simulink model "FRUCD_VehicleSim_Model_V0_1_0"  (R2019b)
settings: Solver=VariableStepAuto  StartTime=0.0  StopTime=7.5  MaxStep=0.001  RelTol=1e-3
undefined symbols (not defined in the file): Alpha, Event, Kappa, Model, Parameter
settings Model: NumberOfSteps=2  Creator=bechr  LastModifiedBy=bechr
settings DebuggingCC: AllowedUnitSystems=CGS,SI,SI (extended)  UnderSpecifiedDimensionMsg=error
settings SFSimCC: CustomCodeUndefinedFunction=UseInterfaceOnly

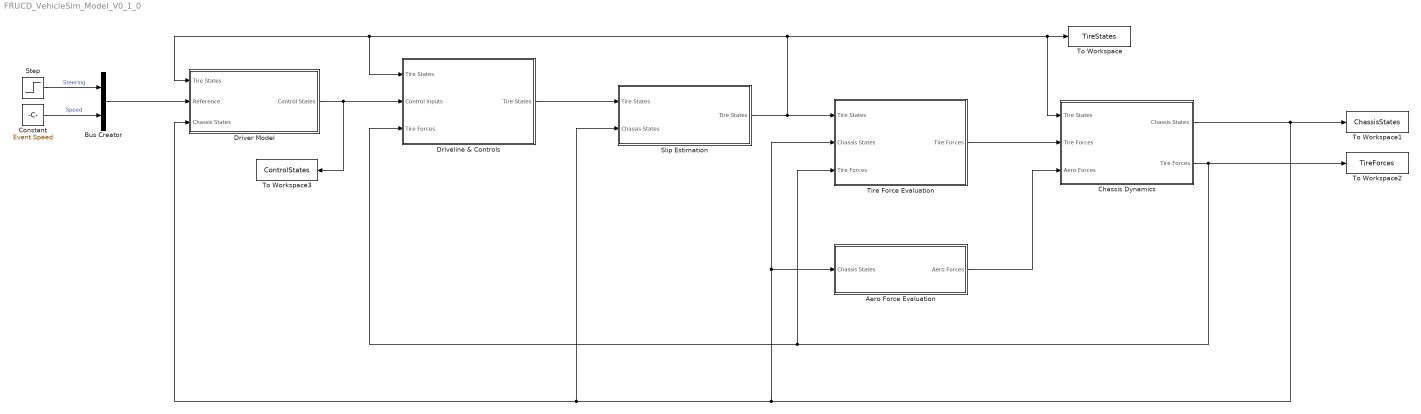
== system FRUCD_VehicleSim_Model_V0_1_0 ==
  Aero Force Evaluation : Subsystem
  Bus Creator : BusCreator  Inputs=2
  Chassis Dynamics : Subsystem  Variant=on
  Constant : Constant  Value=Event.Speed
  Driveline & Controls : Subsystem
  Driver Model : Subsystem  Variant=on
  Slip Estimation : Subsystem  Variant=on
  Step : Step  Time=0.2  After=Event.Amplitude  SampleTime=0
  Tire Force Evaluation : Subsystem
  To Workspace : ToWorkspace  VariableName=TireStates  SaveFormat=Timeseries  SampleTime=-1
  To Workspace1 : ToWorkspace  VariableName=ChassisStates  SaveFormat=Timeseries  SampleTime=-1
  To Workspace2 : ToWorkspace  VariableName=TireForces  SaveFormat=Timeseries  SampleTime=-1
  To Workspace3 : ToWorkspace  VariableName=ControlStates  SaveFormat=Timeseries  SampleTime=-1
  wires:
  Slip Estimation/1(" Tire States") -> Driver Model/1(Tire States), Driveline & Controls/1("Tire States "), To Workspace/1, Chassis Dynamics/1(Tire States), Tire Force Evaluation/1(Tire States)
  Driveline & Controls/1(Tire States) -> Slip Estimation/1(Tire States)
  Tire Force Evaluation/1(" Tire Forces") -> Chassis Dynamics/2("Tire Forces ")
  Chassis Dynamics/1(Chassis States) -> To Workspace1/1, Driver Model/3(Chassis States), Slip Estimation/2(Chassis States), Aero Force Evaluation/1(Chassis States), Tire Force Evaluation/2(Chassis States)
  Aero Force Evaluation/1(Aero Forces) -> Chassis Dynamics/3(Aero Forces)
  Driver Model/1(Control States) -> To Workspace3/1, Driveline & Controls/2(Control Inputs)
  Chassis Dynamics/2(" Tire Forces") -> To Workspace2/1, Driveline & Controls/3(Tire Forces), Tire Force Evaluation/3(Tire Forces)
  Step/1 -> Bus Creator/1  "Steering"
  Constant/1 -> Bus Creator/2  "Speed"
  Bus Creator/1 -> Driver Model/2(Reference)

== system FRUCD_VehicleSim_Model_V0_1_0/Aero Force Evaluation ==
  Chassis States : Inport
  Constant : Constant  Value=[0 0 0 0 0 0]
  Terminator : Terminator
  Aero Forces : Outport
  wires:
  Constant/1 -> Aero Forces/1
  Chassis States/1 -> Terminator/1

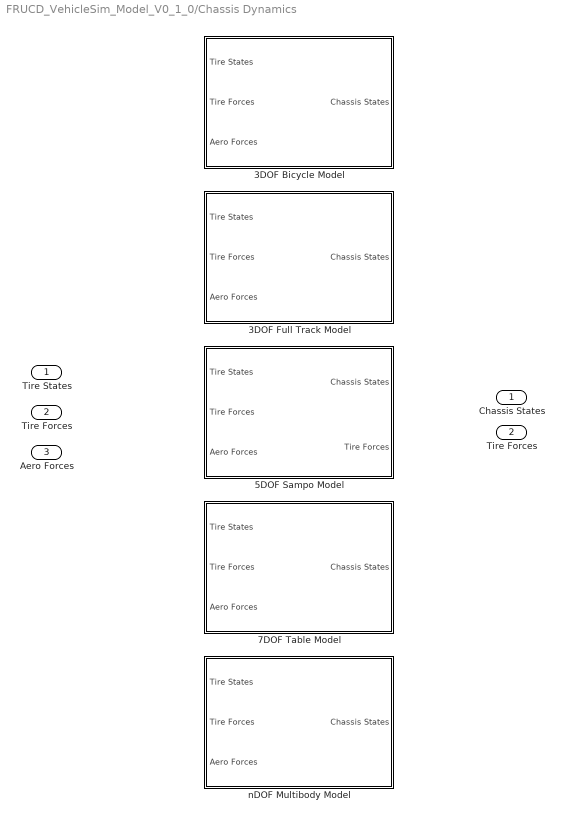
== system FRUCD_VehicleSim_Model_V0_1_0/Chassis Dynamics ==
  Tire States : Inport
  "Tire Forces " : Inport  Port=2
  Aero Forces : Inport  Port=3
  3DOF Bicycle Model : Subsystem  VariantControl="strcmp(Model.ChassisDynamics,\"3DOF Bicycle\")"
  3DOF Full Track Model : Subsystem  VariantControl="strcmp(Model.ChassisDynamics,\"3DOF Full Track\")"
  5DOF Sampo Model : Subsystem  VariantControl="strcmp(Model.ChassisDynamics,\"5DOF Sampo\")"
  "7DOF Table Model " : Subsystem  VariantControl="strcmp(Model.ChassisDynamics,\"7DOF Table\")"
  nDOF Multibody Model : Subsystem  VariantControl="strcmp(Model.ChassisDynamics,\"nDOF Multibody\")"
  Chassis States : Outport
  " Tire Forces" : Outport  Port=2

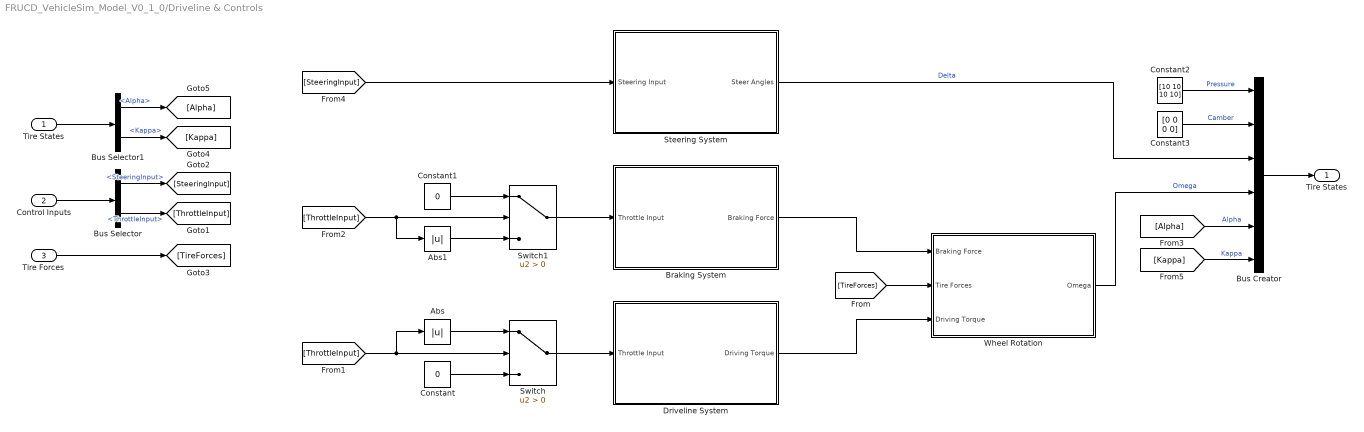
== system FRUCD_VehicleSim_Model_V0_1_0/Driveline & Controls ==
  "Tire States " : Inport
  Control Inputs : Inport  Port=2
  Tire Forces : Inport  Port=3
  Abs : Abs
  Abs1 : Abs
  Braking System : Subsystem  Variant=on
  Bus Creator : BusCreator  Inputs=6
  Bus Selector : BusSelector  OutputSignals=SteeringInput,ThrottleInput
  Bus Selector1 : BusSelector  OutputSignals=Alpha,Kappa
  Constant : Constant  Value=0
  Constant1 : Constant  Value=0
  Constant2 : Constant  Value=[10 10 10 10]
  Constant3 : Constant  Value=[0 0 0 0]
  Driveline System : Subsystem  Variant=on
  Steering System : Subsystem  Variant=on
  Switch : Switch  Criteria=u2 > Threshold
  Switch1 : Switch  Criteria=u2 > Threshold
  Wheel Rotation : Subsystem  Variant=on
  Tire States : Outport
  wires:
  Braking System/1(Braking Force) -> Wheel Rotation/1(Braking Force)
  Driveline System/1(Driving Torque) -> Wheel Rotation/3(Driving Torque)
  Tire Forces/1 -> [TireForces]
  [TireForces] -> Wheel Rotation/2(Tire Forces)
  Control Inputs/1 -> Bus Selector/1
  Bus Selector/1 -> [SteeringInput]  "<SteeringInput>"
  Bus Selector/2 -> [ThrottleInput]  "<ThrottleInput>"
  [ThrottleInput] -> Switch/2, Abs/1
  Switch/1 -> Driveline System/1(Throttle Input)
  Constant/1 -> Switch/3
  Abs/1 -> Switch/1
  Switch1/1 -> Braking System/1(Throttle Input)
  [ThrottleInput] -> Abs1/1, Switch1/2
  Constant1/1 -> Switch1/1
  Abs1/1 -> Switch1/3
  Bus Creator/1 -> Tire States/1
  Constant2/1 -> Bus Creator/1  "Pressure"
  Constant3/1 -> Bus Creator/2  "Camber"
  Wheel Rotation/1(Omega) -> Bus Creator/4  "Omega"
  Steering System/1(Steer Angles) -> Bus Creator/3  "Delta"
  [SteeringInput] -> Steering System/1(Steering Input)
  Bus Selector1/1 -> [Alpha]  "<Alpha>"
  Bus Selector1/2 -> [Kappa]  "<Kappa>"
  "Tire States "/1 -> Bus Selector1/1
  [Alpha] -> Bus Creator/5  "Alpha"
  [Kappa] -> Bus Creator/6  "Kappa"

== system FRUCD_VehicleSim_Model_V0_1_0/Driver Model ==
  Tire States : Inport
  Reference : Inport  Port=2
  Chassis States : Inport  Port=3
  MPC Path Following : Subsystem  VariantControl="strcmp(Model.Driver,\"Path Following\")"
  Open Loop Steer & Speed Regulation : Subsystem  VariantControl="strcmp(Model.Driver,\"Open Loop & Regulation Control\")"
  Control States : Outport

== system FRUCD_VehicleSim_Model_V0_1_0/Slip Estimation ==
  Tire States : Inport
  Chassis States : Inport  Port=2
  Full Fidelity : Subsystem  VariantControl="strcmp(Model.SlipEstimation,\"Full Fidelity\")"
  Planar Geometry : Subsystem  VariantControl="strcmp(Model.SlipEstimation,\"Planar\")"
  " Tire States" : Outport

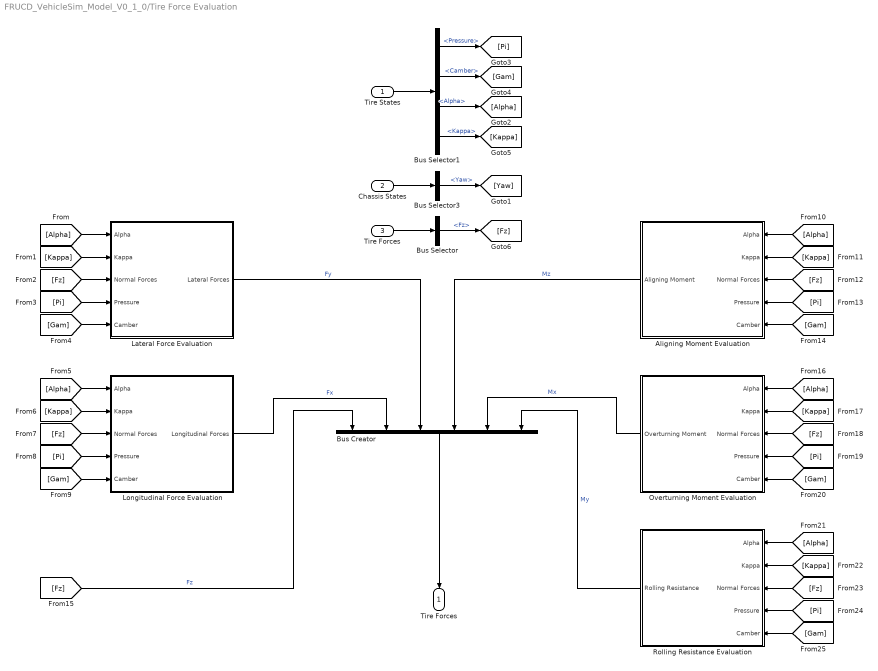
== system FRUCD_VehicleSim_Model_V0_1_0/Tire Force Evaluation ==
  Tire States : Inport
  Chassis States : Inport  Port=2
  Tire Forces : Inport  Port=3
  Aligning Moment Evaluation : Subsystem  Variant=on
  Bus Creator : BusCreator  Inputs=6
  Bus Selector : BusSelector  OutputSignals=Fz
  Bus Selector1 : BusSelector  OutputSignals=Pressure,Camber,Alpha,Kappa
  Bus Selector3 : BusSelector  OutputSignals=Vel.Yaw
  Lateral Force Evaluation : Subsystem  Variant=on
  Longitudinal Force Evaluation : Subsystem  Variant=on
  Overturning Moment Evaluation : Subsystem  Variant=on
  Rolling Resistance Evaluation : Subsystem  Variant=on
  " Tire Forces" : Outport  VectorParamsAs1DForOutWhenUnconnected=off
  wires:
  [Pi] -> Lateral Force Evaluation/4(Pressure)
  Bus Creator/1 -> " Tire Forces"/1
  Aligning Moment Evaluation/1(Aligning Moment) -> Bus Creator/4  "Mz"
  [Alpha] -> Aligning Moment Evaluation/1(Alpha)
  Rolling Resistance Evaluation/1(Rolling Resistance) -> Bus Creator/6  "My"
  [Fz] -> Bus Creator/1  "Fz"
  Longitudinal Force Evaluation/1(Longitudinal Forces) -> Bus Creator/2  "Fx"
  [Fz] -> Rolling Resistance Evaluation/3(Normal Forces)
  [Kappa] -> Longitudinal Force Evaluation/2(Kappa)
  [Pi] -> Rolling Resistance Evaluation/4(Pressure)
  [Gam] -> Overturning Moment Evaluation/5(Camber)
  Overturning Moment Evaluation/1(Overturning Moment) -> Bus Creator/5  "Mx"
  [Kappa] -> Lateral Force Evaluation/2(Kappa)
  Lateral Force Evaluation/1(Lateral Forces) -> Bus Creator/3  "Fy"
  [Kappa] -> Rolling Resistance Evaluation/2(Kappa)
  [Alpha] -> Lateral Force Evaluation/1(Alpha)
  [Gam] -> Rolling Resistance Evaluation/5(Camber)
  [Fz] -> Lateral Force Evaluation/3(Normal Forces)
  [Fz] -> Aligning Moment Evaluation/3(Normal Forces)
  [Fz] -> Overturning Moment Evaluation/3(Normal Forces)
  [Pi] -> Longitudinal Force Evaluation/4(Pressure)
  [Pi] -> Overturning Moment Evaluation/4(Pressure)
  [Alpha] -> Overturning Moment Evaluation/1(Alpha)
  [Kappa] -> Overturning Moment Evaluation/2(Kappa)
  [Pi] -> Aligning Moment Evaluation/4(Pressure)
  [Gam] -> Lateral Force Evaluation/5(Camber)
  [Alpha] -> Longitudinal Force Evaluation/1(Alpha)
  [Kappa] -> Aligning Moment Evaluation/2(Kappa)
  [Gam] -> Aligning Moment Evaluation/5(Camber)
  [Fz] -> Longitudinal Force Evaluation/3(Normal Forces)
  [Gam] -> Longitudinal Force Evaluation/5(Camber)
  [Alpha] -> Rolling Resistance Evaluation/1(Alpha)
  Tire Forces/1 -> Bus Selector/1
  Bus Selector/1 -> [Fz]  "<Fz>"
  Tire States/1 -> Bus Selector1/1
  Bus Selector1/2 -> [Gam]  "<Camber>"
  Bus Selector1/1 -> [Pi]  "<Pressure>"
  Chassis States/1 -> Bus Selector3/1
  Bus Selector3/1 -> [Yaw]  "<Yaw>"
  Bus Selector1/3 -> [Alpha]  "<Alpha>"
  Bus Selector1/4 -> [Kappa]  "<Kappa>"

== system FRUCD_VehicleSim_Model_V0_1_0/Chassis Dynamics/3DOF Bicycle Model ==
  Tire States : Inport
  "Tire Forces " : Inport  Port=2
  Aero Forces : Inport  Port=3
  Chassis States : Outport

== system FRUCD_VehicleSim_Model_V0_1_0/Chassis Dynamics/3DOF Full Track Model ==
  Tire States : Inport
  "Tire Forces " : Inport  Port=2
  Aero Forces : Inport  Port=3
  Chassis States : Outport

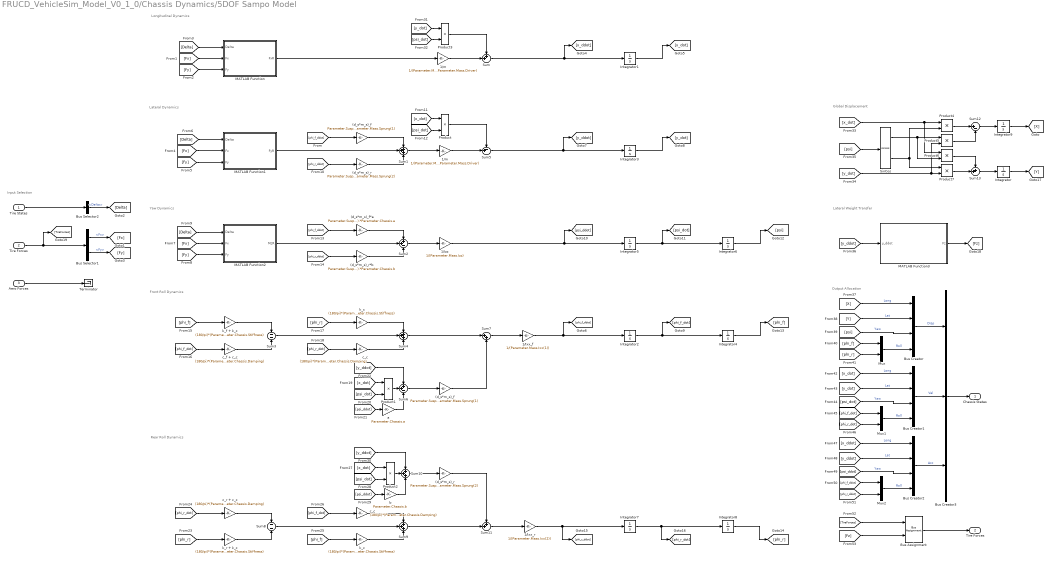
== system FRUCD_VehicleSim_Model_V0_1_0/Chassis Dynamics/5DOF Sampo Model ==
  note: Output Allocation
  note: Lateral Weight Transfer
  note: Global Displacement
  note: Input Selection
  note: Rear Roll Dynamics
  note: Front Roll Dynamics
  note: Yaw Dynamics
  note: Lateral Dynamics
  note: Longitudinal Dynamics
  Tire States : Inport
  "Tire Forces " : Inport  Port=2
  Aero Forces : Inport  Port=3
  (d_s*m_s)_f : Gain  Gain=Parameter.Suspension.Roll.Arm(1).*Parameter.Mass.Sprung(1)
  "(d_s*m_s)_f " : Gain  Gain=Parameter.Suspension.Roll.Arm(1).*Parameter.Mass.Sprung(1)
  (d_s*m_s)_f*a : Gain  Gain=Parameter.Suspension.Roll.Arm(1).*Parameter.Mass.Sprung(1).*Parameter.Chassis.a
  (d_s*m_s)_r : Gain  Gain=Parameter.Suspension.Roll.Arm(2).*Parameter.Mass.Sprung(2)
  "(d_s*m_s)_r " : Gain  Gain=Parameter.Suspension.Roll.Arm(2).*Parameter.Mass.Sprung(2)
  (d_s*m_s)_r*b : Gain  Gain=Parameter.Suspension.Roll.Arm(2).*Parameter.Mass.Sprung(2).*Parameter.Chassis.b
  1/Ixx_f : Gain  Gain=1/(Parameter.Mass.Ixx(1))
  1/Ixx_r : Gain  Gain=1/(Parameter.Mass.Ixx(2))
  1/Izz : Gain  Gain=1/(Parameter.Mass.Izz)
  1/m : Gain  Gain=1/(Parameter.Mass.Vehicle+Parameter.Mass.Driver)
  "1/m " : Gain  Gain=1/(Parameter.Mass.Vehicle+Parameter.Mass.Driver)
  Bus Assignment : BusAssignment  AssignedSignals=Fz
  Bus Creator : BusCreator  Inputs=4
  Bus Creator1 : BusCreator  Inputs=4
  Bus Creator2 : BusCreator  Inputs=4
  Bus Creator3 : BusCreator  Inputs=3
  Bus Selector1 : BusSelector  OutputSignals=Fx,Fy
  Bus Selector2 : BusSelector  OutputSignals=Delta
  Integrator{,2..9} (9 alike) : Integrator
  Integrator1 : Integrator  InitialCondition=Event.Speed
  MATLAB Function : MATLAB Function  TreatAsAtomicUnit=on
  MATLAB Function1 : MATLAB Function  TreatAsAtomicUnit=on
  MATLAB Function2 : MATLAB Function  TreatAsAtomicUnit=on
  MATLAB Function3 : MATLAB Function  TreatAsAtomicUnit=on
  Mux : Mux  Inputs=2
  Mux1 : Mux  Inputs=2
  Mux2 : Mux  Inputs=2
  Product{,1..7} (8 alike) : Product
  SinCos : Trigonometry  Operator=sincos
  Sum : Sum  Inputs=++|
  Sum{1,4,9..10} (4 alike) : Sum  Inputs=+++
  Sum11 : Sum  Inputs=++|
  Sum12 : Sum  Inputs=|+-
  Sum13 : Sum  Inputs=++|
  Sum2 : Sum  Inputs=++-
  Sum3 : Sum  Inputs=-|-
  Sum5 : Sum  Inputs=-+|
  Sum6 : Sum  Inputs=++-
  Sum7 : Sum  Inputs=|++
  Sum8 : Sum  Inputs=-|-
  Terminator : Terminator
  a : Gain  Gain=Parameter.Chassis.a
  b : Gain  Gain=Parameter.Chassis.b
  c_c : Gain  Gain=(180/pi)*(Parameter.Chassis.Damping)
  "c_c " : Gain  Gain=(180/pi)*(Parameter.Chassis.Damping)
  c_f + c_c : Gain  Gain=(180/pi)*(Parameter.Suspension.Roll.Damping(1)+Parameter.Chassis.Damping)
  c_r + c_c : Gain  Gain=(180/pi)*(Parameter.Suspension.Roll.Damping(2)+Parameter.Chassis.Damping)
  k_c : Gain  Gain=(180/pi)*(Parameter.Chassis.Stiffness)
  "k_c " : Gain  Gain=(180/pi)*(Parameter.Chassis.Stiffness)
  k_f + k_c : Gain  Gain=(180/pi)*(Parameter.Suspension.Roll.Stiffness(1)+Parameter.Chassis.Stiffness)
  k_r + k_c : Gain  Gain=(180/pi)*(Parameter.Suspension.Roll.Stiffness(2)+Parameter.Chassis.Stiffness)
  Chassis States : Outport
  " Tire Forces" : Outport  Port=2
  wires:
  Tire States/1 -> Bus Selector2/1
  Bus Selector2/1 -> [Delta]  "<Delta>"
  Bus Selector1/2 -> [Fy]  "<Fy>"
  Bus Selector1/1 -> [Fx]  "<Fx>"
  Aero Forces/1 -> Terminator/1
  Product3/1 -> Sum/1
  c_f + c_c/1 -> Sum3/2
  [psi_dot] -> Product2/2
  "c_c "/1 -> Sum9/1
  Sum6/1 -> "(d_s*m_s)_f "/1
  [psi_dot] -> Product3/2
  b/1 -> Sum10/3
  MATLAB Function1/1(FyR) -> Sum1/2
  Integrator7/1 -> [phi_r_dot], Integrator8/1
  [phi_f_ddot] -> (d_s*m_s)_f*a/1
  Sum7/1 -> 1/Ixx_f/1
  [Delta] -> MATLAB Function1/1(Delta)
  Sum1/1 -> "1/m "/1
  Sum11/1 -> 1/Ixx_r/1
  "(d_s*m_s)_f "/1 -> Sum7/2
  [y_ddot] -> Sum10/1
  [psi_dot] -> Product1/2
  [psi_dot] -> Product/2
  [phi_r] -> k_c/1
  "k_c "/1 -> Sum9/3
  Product2/1 -> Sum10/2
  Sum8/1 -> Sum9/2
  [phi_f_dot] -> c_f + c_c/1
  Product1/1 -> Sum6/2
  [phi_r] -> k_r + k_c/1
  MATLAB Function2/1(MzR) -> Sum2/2
  [Fx] -> MATLAB Function2/2(Fx)
  [phi_f_dot] -> "c_c "/1
  [phi_r_dot] -> c_c/1
  [x_dot] -> Product1/1
  [psi_ddot] -> a/1
  "1/m "/1 -> Sum5/2
  [Fy] -> MATLAB Function2/3(Fy)
  [phi_r_ddot] -> (d_s*m_s)_r*b/1
  1/Izz/1 -> [psi_ddot], Integrator5/1
  [x_dot] -> Product2/1
  Integrator5/1 -> [psi_dot], Integrator6/1
  Integrator4/1 -> [phi_f]
  [phi_f_ddot] -> (d_s*m_s)_f/1
  Sum4/1 -> Sum7/1
  c_r + c_c/1 -> Sum8/1
  [x_dot] -> Product/1
  Sum2/1 -> 1/Izz/1
  [phi_f] -> k_f + k_c/1
  "(d_s*m_s)_r "/1 -> Sum11/1
  Sum9/1 -> Sum11/2
  [y_ddot] -> Sum6/1
  (d_s*m_s)_r/1 -> Sum1/3
  [Fy] -> MATLAB Function/3(Fy)
  Integrator3/1 -> [y_dot]
  Product/1 -> Sum5/1
  Integrator1/1 -> [x_dot]
  MATLAB Function/1(FxR) -> 1/m/1
  1/m/1 -> Sum/2
  (d_s*m_s)_f/1 -> Sum1/1
  Integrator8/1 -> [phi_r]
  (d_s*m_s)_f*a/1 -> Sum2/1
  Sum3/1 -> Sum4/2
  Integrator6/1 -> [psi]
  1/Ixx_r/1 -> [phi_r_ddot], Integrator7/1
  Sum10/1 -> "(d_s*m_s)_r "/1
  Integrator2/1 -> [phi_f_dot], Integrator4/1
  a/1 -> Sum6/3
  k_f + k_c/1 -> Sum3/1
  c_c/1 -> Sum4/3
  1/Ixx_f/1 -> [phi_f_ddot], Integrator2/1
  Sum/1 -> [x_ddot], Integrator1/1
  [psi_ddot] -> b/1
  [y_dot] -> Product3/1
  (d_s*m_s)_r*b/1 -> Sum2/3
  [Fx] -> MATLAB Function1/2(Fx)
  k_c/1 -> Sum4/1
  k_r + k_c/1 -> Sum8/2
  [Delta] -> MATLAB Function/1(Delta)
  Sum5/1 -> [y_ddot], Integrator3/1
  [Fx] -> MATLAB Function/2(Fx)
  [phi_r_ddot] -> (d_s*m_s)_r/1
  [phi_f] -> "k_c "/1
  [Fy] -> MATLAB Function1/3(Fy)
  [phi_r_dot] -> c_r + c_c/1
  [Delta] -> MATLAB Function2/1(Delta)
  [x_dot] -> Product4/1, Product6/1
  [y_dot] -> Product5/2, Product7/2
  SinCos/1 -> Product6/2, Product5/1
  SinCos/2 -> Product7/1, Product4/2
  Product4/1 -> Sum12/1
  Product5/1 -> Sum12/2
  Product6/1 -> Sum13/1
  Product7/1 -> Sum13/2
  Sum13/1 -> Integrator/1
  Sum12/1 -> Integrator9/1
  Integrator9/1 -> [X]
  Integrator/1 -> [Y]
  [y_ddot] -> MATLAB Function3/1(y_ddot)
  MATLAB Function3/1(Fz) -> [Fz]
  [phi_f] -> Mux/1
  [phi_r] -> Mux/2
  [X] -> Bus Creator/1  "Long"
  [Y] -> Bus Creator/2  "Lat"
  [psi] -> Bus Creator/3  "Yaw"
  Mux/1 -> Bus Creator/4  "Roll"
  [phi_f_dot] -> Mux1/1
  [psi_dot] -> Bus Creator1/3  "Yaw"
  [phi_r_dot] -> Mux1/2
  [y_dot] -> Bus Creator1/2  "Lat"
  Mux1/1 -> Bus Creator1/4  "Roll"
  [x_dot] -> Bus Creator1/1  "Long"
  [psi_ddot] -> Bus Creator2/3  "Yaw"
  [phi_r_ddot] -> Mux2/2
  [phi_f_ddot] -> Mux2/1
  [x_ddot] -> Bus Creator2/1  "Long"
  Mux2/1 -> Bus Creator2/4  "Roll"
  [y_ddot] -> Bus Creator2/2  "Lat"
  Bus Creator2/1 -> Bus Creator3/3  "Acc"
  Bus Creator1/1 -> Bus Creator3/2  "Vel"
  Bus Creator/1 -> Bus Creator3/1  "Disp"
  Bus Creator3/1 -> Chassis States/1
  "Tire Forces "/1 -> [TireForces], Bus Selector1/1
  [TireForces] -> Bus Assignment/1
  [Fz] -> Bus Assignment/2
  Bus Assignment/1 -> " Tire Forces"/1
  [psi] -> SinCos/1

== system FRUCD_VehicleSim_Model_V0_1_0/Chassis Dynamics/7DOF Table Model  ==
  Tire States : Inport
  "Tire Forces " : Inport  Port=2
  Aero Forces : Inport  Port=3
  Chassis States : Outport

== system FRUCD_VehicleSim_Model_V0_1_0/Chassis Dynamics/nDOF Multibody Model ==
  Tire States : Inport
  "Tire Forces " : Inport  Port=2
  Aero Forces : Inport  Port=3
  Chassis States : Outport

== system FRUCD_VehicleSim_Model_V0_1_0/Driveline & Controls/Braking System ==
  Throttle Input : Inport
  Bond Graph Model : Subsystem  VariantControl="strcmp(Model.BrakingSystem,\"Bond Graph Model\")"
  Linear Gains : Subsystem  VariantControl="strcmp(Model.BrakingSystem,\"Simple Gains\")"
  Braking Force : Outport

== system FRUCD_VehicleSim_Model_V0_1_0/Driveline & Controls/Driveline System ==
  Throttle Input : Inport
  Bond Graph : Subsystem  VariantControl="strcmp(Model.DrivelineSystem,\"Bond Graph Model\")"
  Linear Gains : Subsystem  VariantControl="strcmp(Model.DrivelineSystem,\"Simple Gains\")"
  Driving Torque : Outport

== system FRUCD_VehicleSim_Model_V0_1_0/Driveline & Controls/Steering System ==
  Steering Input : Inport
  Ackermann Lookup : Subsystem  VariantControl="strcmp(Model.SteeringSystem,\"Lookup Table\")"
  Linear Gain : Subsystem  VariantControl="strcmp(Model.SteeringSystem,\"Simple Gains\")"
  Steer Angles : Outport

== system FRUCD_VehicleSim_Model_V0_1_0/Driveline & Controls/Wheel Rotation ==
  Braking Force : Inport
  Tire Forces : Inport  Port=2
  Driving Torque : Inport  Port=3
  Simple ODE : Subsystem  VariantControl="strcmp(Model.WheelRotation,\"Simple ODE\")"
  Omega : Outport

== system FRUCD_VehicleSim_Model_V0_1_0/Driver Model/MPC Path Following ==
  Tire States : Inport
  Reference : Inport  Port=2
  Chassis States : Inport  Port=3
  Control States : Outport

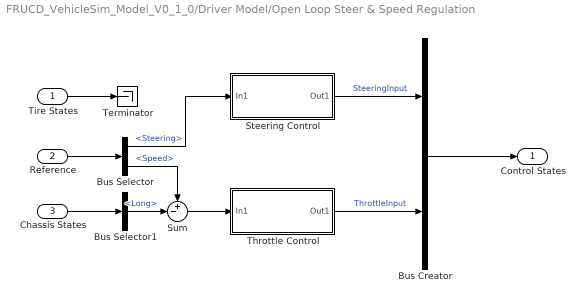
== system FRUCD_VehicleSim_Model_V0_1_0/Driver Model/Open Loop Steer & Speed Regulation ==
  Tire States : Inport
  Reference : Inport  Port=2
  Chassis States : Inport  Port=3
  Bus Creator : BusCreator  Inputs=2
  Bus Selector : BusSelector  OutputSignals=Steering,Speed
  Bus Selector1 : BusSelector  OutputSignals=Vel.Long
  Steering Control : Subsystem
  Sum : Sum  Inputs=+-|
  Terminator : Terminator
  Throttle Control : Subsystem
  Control States : Outport
  wires:
  Reference/1 -> Bus Selector/1
  Tire States/1 -> Terminator/1
  Chassis States/1 -> Bus Selector1/1
  Steering Control/1(Out1) -> Bus Creator/1  "SteeringInput"
  Throttle Control/1(Out1) -> Bus Creator/2  "ThrottleInput"
  Bus Creator/1 -> Control States/1
  Bus Selector/1 -> Steering Control/1(In1)  "<Steering>"
  Bus Selector/2 -> Sum/1  "<Speed>"
  Bus Selector1/1 -> Sum/2  "<Long>"
  Sum/1 -> Throttle Control/1(In1)

== system FRUCD_VehicleSim_Model_V0_1_0/Slip Estimation/Full Fidelity ==
  Chassis States : Inport
  Tire States : Inport  Port=2
  " Tire States" : Outport

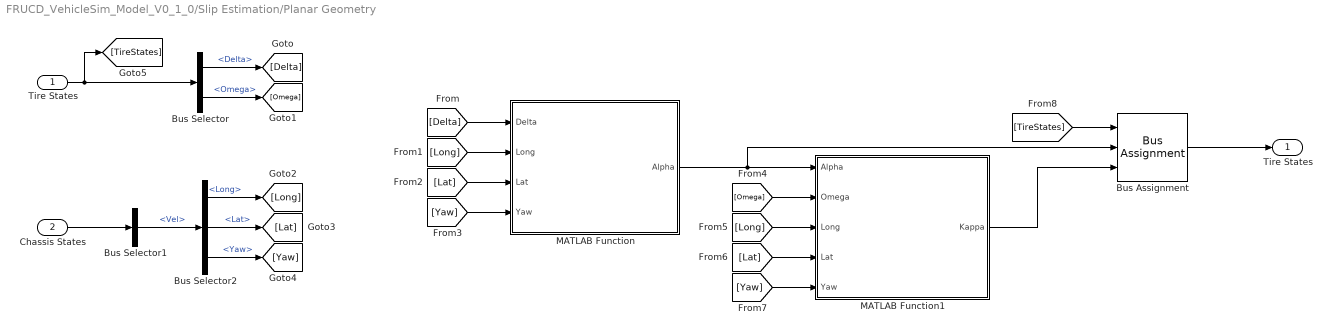
== system FRUCD_VehicleSim_Model_V0_1_0/Slip Estimation/Planar Geometry ==
  Tire States : Inport
  Chassis States : Inport  Port=2
  Bus Assignment : BusAssignment  AssignedSignals=Alpha,Kappa
  Bus Selector : BusSelector  OutputSignals=Delta,Omega
  Bus Selector1 : BusSelector  OutputSignals=Vel
  Bus Selector2 : BusSelector  OutputSignals=Long,Lat,Yaw
  MATLAB Function : MATLAB Function  TreatAsAtomicUnit=on
  MATLAB Function1 : MATLAB Function  TreatAsAtomicUnit=on
  " Tire States" : Outport
  wires:
  [Yaw] -> MATLAB Function/4(Yaw)
  [Lat] -> MATLAB Function/3(Lat)
  [Long] -> MATLAB Function/2(Long)
  [Delta] -> MATLAB Function/1(Delta)
  Tire States/1 -> [TireStates], Bus Selector/1
  [Yaw] -> MATLAB Function1/5(Yaw)
  [Lat] -> MATLAB Function1/4(Lat)
  [Long] -> MATLAB Function1/3(Long)
  [Omega] -> MATLAB Function1/2(Omega)
  MATLAB Function/1(Alpha) -> Bus Assignment/2, MATLAB Function1/1(Alpha)
  Bus Selector/1 -> [Delta]  "<Delta>"
  Bus Selector/2 -> [Omega]  "<Omega>"
  Chassis States/1 -> Bus Selector1/1
  [TireStates] -> Bus Assignment/1
  Bus Assignment/1 -> " Tire States"/1
  Bus Selector1/1 -> Bus Selector2/1  "<Vel>"
  Bus Selector2/1 -> [Long]  "<Long>"
  Bus Selector2/2 -> [Lat]  "<Lat>"
  Bus Selector2/3 -> [Yaw]  "<Yaw>"
  MATLAB Function1/1(Kappa) -> Bus Assignment/3

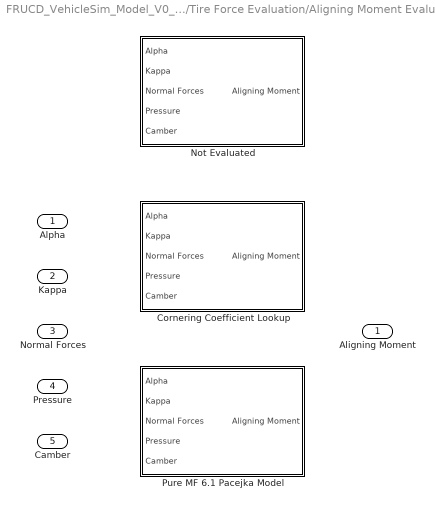
== system FRUCD_VehicleSim_Model_V0_1_0/Tire Force Evaluation/Aligning Moment Evaluation ==
  Alpha : Inport
  Kappa : Inport  Port=2
  Normal Forces : Inport  Port=3
  Pressure : Inport  Port=4
  Camber : Inport  Port=5
  Cornering Coefficient Lookup : Subsystem  VariantControl="strcmp(Model.TireForceEvaluation.Aligning,\"Cornering Coefficient\")"
  Not Evaluated : Subsystem  VariantControl="strcmp(Model.TireForceEvaluation.Aligning,\"Not Evaluated\")"
  Pure MF 6.1 Pacejka Model : Subsystem  VariantControl="strcmp(Model.TireForceEvaluation.Aligning,\"Pure MF6.1\")"
  Aligning Moment : Outport  VectorParamsAs1DForOutWhenUnconnected=off

== system FRUCD_VehicleSim_Model_V0_1_0/Tire Force Evaluation/Lateral Force Evaluation ==
  Alpha : Inport
  Kappa : Inport  Port=2
  Normal Forces : Inport  Port=3
  Pressure : Inport  Port=4
  Camber : Inport  Port=5
  Cornering Coefficient Lookup : Subsystem  VariantControl="strcmp(Model.TireForceEvaluation.Lateral,\"Cornering Coefficient\")"
  Pure MF 6.1 Pacejka Model : Subsystem  VariantControl="strcmp(Model.TireForceEvaluation.Lateral,\"Pure MF6.1\")"
  Lateral Forces : Outport  VectorParamsAs1DForOutWhenUnconnected=off

== system FRUCD_VehicleSim_Model_V0_1_0/Tire Force Evaluation/Longitudinal Force Evaluation ==
  Alpha : Inport
  Kappa : Inport  Port=2
  Normal Forces : Inport  Port=3
  Pressure : Inport  Port=4
  Camber : Inport  Port=5
  Cornering Coefficient Lookup : Subsystem  VariantControl="strcmp(Model.TireForceEvaluation.Longitudinal,\"Cornering Coefficient\")"
  Pure MF 6.1 Pacejka Model : Subsystem  VariantControl="strcmp(Model.TireForceEvaluation.Longitudinal,\"Pure MF6.1\")"
  Longitudinal Forces : Outport  VectorParamsAs1DForOutWhenUnconnected=off

== system FRUCD_VehicleSim_Model_V0_1_0/Tire Force Evaluation/Overturning Moment Evaluation ==
  Alpha : Inport
  Kappa : Inport  Port=2
  Normal Forces : Inport  Port=3
  Pressure : Inport  Port=4
  Camber : Inport  Port=5
  Cornering Coefficient Lookup : Subsystem  VariantControl="strcmp(Model.TireForceEvaluation.Overturning,\"Cornering Coefficient\")"
  Not Evaluated : Subsystem  VariantControl="strcmp(Model.TireForceEvaluation.Overturning,\"Not Evaluated\")"
  Pure MF 6.1 Pacejka Model : Subsystem  VariantControl="strcmp(Model.TireForceEvaluation.Overturning,\"Pure MF6.1\")"
  Overturning Moment : Outport  VectorParamsAs1DForOutWhenUnconnected=off

== system FRUCD_VehicleSim_Model_V0_1_0/Tire Force Evaluation/Rolling Resistance Evaluation ==
  Alpha : Inport
  Kappa : Inport  Port=2
  Normal Forces : Inport  Port=3
  Pressure : Inport  Port=4
  Camber : Inport  Port=5
  Cornering Coefficient Lookup : Subsystem  VariantControl="strcmp(Model.TireForceEvaluation.Rolling,\"Cornering Coefficient\")"
  Not Evaluated : Subsystem  VariantControl="strcmp(Model.TireForceEvaluation.Overturning,\"Not Evaluated\")"
  Pure MF 6.1 Pacejka Model : Subsystem  VariantControl="strcmp(Model.TireForceEvaluation.Rolling,\"Pure MF6.1\")"
  Rolling Resistance : Outport  VectorParamsAs1DForOutWhenUnconnected=off

== system FRUCD_VehicleSim_Model_V0_1_0/Driveline & Controls/Braking System/Bond Graph Model ==
  Throttle Input : Inport
  Braking Force : Outport

== system FRUCD_VehicleSim_Model_V0_1_0/Driveline & Controls/Braking System/Linear Gains ==
  Throttle Input : Inport
  Friction Coefficient [ ] : Gain  Gain=Parameter.Brake.Pad.Mu
  Front Bore Area [m^2] : Gain  Gain=1 / (pi*Parameter.Brake.Cylinder.Bore(1)^2)
  Mux : Mux
  Pad Area [m^2] * Pad Quantity [ ] : Gain  Gain=Parameter.Brake.Pad.No*Parameter.Brake.Pad.Area
  Pedal Force [N] : Gain  Gain=Parameter.Brake.Pedal.Force
  Pedal Ratio [ ] : Gain  Gain=Parameter.Brake.Pedal.Ratio
  Rear Bore Area [m^2] : Gain  Gain=1 / (pi*Parameter.Brake.Cylinder.Bore(2)^2)
  Braking Force : Outport
  wires:
  Throttle Input/1 -> Pedal Force [N]/1
  Pedal Force [N]/1 -> Pedal Ratio [ ]/1
  Front Bore Area [m^2]/1 -> Mux/1, Mux/2
  Rear Bore Area [m^2]/1 -> Mux/3, Mux/4
  Mux/1 -> Pad Area [m^2] * Pad Quantity [ ]/1
  Pad Area [m^2] * Pad Quantity [ ]/1 -> Friction Coefficient [ ]/1
  Friction Coefficient [ ]/1 -> Braking Force/1
  Pedal Ratio [ ]/1 -> Front Bore Area [m^2]/1, Rear Bore Area [m^2]/1

== system FRUCD_VehicleSim_Model_V0_1_0/Driveline & Controls/Driveline System/Bond Graph ==
  Throttle Input : Inport
  Driving Torque : Outport

== system FRUCD_VehicleSim_Model_V0_1_0/Driveline & Controls/Driveline System/Linear Gains ==
  Throttle Input : Inport
  Constant : Constant  Value=0
  Maximum Torque [Nm] : Gain  Gain=157/2
  Mux : Mux
  Driving Torque : Outport
  wires:
  Throttle Input/1 -> Maximum Torque [Nm]/1
  Constant/1 -> Mux/2, Mux/1
  Maximum Torque [Nm]/1 -> Mux/4, Mux/3
  Mux/1 -> Driving Torque/1

== system FRUCD_VehicleSim_Model_V0_1_0/Driveline & Controls/Steering System/Ackermann Lookup ==
  Steering Input : Inport
  Steer Angles : Outport

== system FRUCD_VehicleSim_Model_V0_1_0/Driveline & Controls/Steering System/Linear Gain ==
  Steering Input : Inport
  Ackermann Lookup : Lookup_n-D  NumberOfTableDimensions=1  BreakpointsForDimension1=linspace(-120,120,20)  Table=linspace(-30,30,20)  InterpMethod=Cubic spline  InternalRulePriority=Speed  RndMeth=Simplest  InputSameDT=on
  Constant : Constant  Value=0
  Max Steering Angle [deg] : Gain  Gain=120
  Mux : Mux
  Steer Angles : Outport
  wires:
  Steering Input/1 -> Max Steering Angle [deg]/1
  Max Steering Angle [deg]/1 -> Ackermann Lookup/1
  Mux/1 -> Steer Angles/1
  Constant/1 -> Mux/4, Mux/3
  Ackermann Lookup/1 -> Mux/2, Mux/1

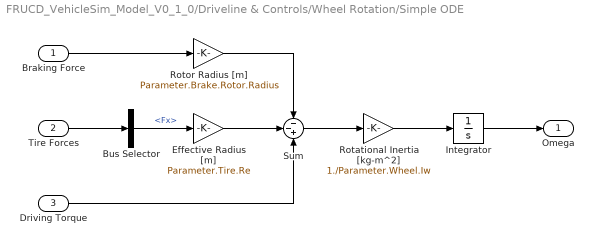
== system FRUCD_VehicleSim_Model_V0_1_0/Driveline & Controls/Wheel Rotation/Simple ODE ==
  Braking Force : Inport
  Tire Forces : Inport  Port=2
  Driving Torque : Inport  Port=3
  Bus Selector : BusSelector  OutputSignals=Fx
  Effective Radius [m] : Gain  Gain=Parameter.Tire.Re
  Integrator : Integrator  InitialCondition=Event.Speed/Parameter.Tire.Re.*ones(4,1)
  Rotational Inertia [kg-m^2] : Gain  Gain=1./Parameter.Wheel.Iw
  Rotor Radius [m] : Gain  Gain=Parameter.Brake.Rotor.Radius
  Sum : Sum  Inputs=--+
  Omega : Outport
  wires:
  Tire Forces/1 -> Bus Selector/1
  Effective Radius [m]/1 -> Sum/2
  Rotor Radius [m]/1 -> Sum/1
  Bus Selector/1 -> Effective Radius [m]/1  "<Fx>"
  Sum/1 -> Rotational Inertia [kg-m^2]/1
  Rotational Inertia [kg-m^2]/1 -> Integrator/1
  Integrator/1 -> Omega/1
  Braking Force/1 -> Rotor Radius [m]/1
  Driving Torque/1 -> Sum/3

== system FRUCD_VehicleSim_Model_V0_1_0/Driver Model/Open Loop Steer & Speed Regulation/Steering Control ==
  In1 : Inport
  Out1 : Outport
  wires:
  In1/1 -> Out1/1

== system FRUCD_VehicleSim_Model_V0_1_0/Driver Model/Open Loop Steer & Speed Regulation/Throttle Control ==
  In1 : Inport
  Saturation : Saturate  UpperLimit=1  LowerLimit=-1
  Out1 : Outport
  wires:
  Saturation/1 -> Out1/1
  In1/1 -> Saturation/1

== system FRUCD_VehicleSim_Model_V0_1_0/Tire Force Evaluation/Aligning Moment Evaluation/Cornering Coefficient Lookup ==
  Alpha : Inport
  Kappa : Inport  Port=2
  Normal Forces : Inport  Port=3
  Pressure : Inport  Port=4
  Camber : Inport  Port=5
  MATLAB Function : MATLAB Function  TreatAsAtomicUnit=on
  Aligning Moment : Outport  VectorParamsAs1DForOutWhenUnconnected=off
  wires:
  Camber/1 -> MATLAB Function/5(Gam)
  Pressure/1 -> MATLAB Function/4(Pi)
  Normal Forces/1 -> MATLAB Function/3(Fz)
  Kappa/1 -> MATLAB Function/2(unused)
  Alpha/1 -> MATLAB Function/1(a)
  MATLAB Function/1(Fyo) -> Aligning Moment/1

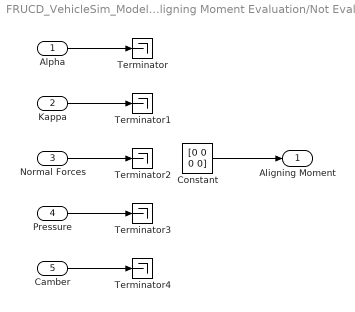
== system FRUCD_VehicleSim_Model_V0_1_0/Tire Force Evaluation/Aligning Moment Evaluation/Not Evaluated ==
  Alpha : Inport
  Kappa : Inport  Port=2
  Normal Forces : Inport  Port=3
  Pressure : Inport  Port=4
  Camber : Inport  Port=5
  Constant : Constant  Value=[0 0 0 0]
  Terminator{,1..4} (5 alike) : Terminator
  Aligning Moment : Outport  VectorParamsAs1DForOutWhenUnconnected=off
  wires:
  Kappa/1 -> Terminator1/1
  Alpha/1 -> Terminator/1
  Constant/1 -> Aligning Moment/1
  Normal Forces/1 -> Terminator2/1
  Pressure/1 -> Terminator3/1
  Camber/1 -> Terminator4/1

== system FRUCD_VehicleSim_Model_V0_1_0/Tire Force Evaluation/Aligning Moment Evaluation/Pure MF 6.1 Pacejka Model ==
  Alpha : Inport
  Kappa : Inport  Port=2
  Normal Forces : Inport  Port=3
  Pressure : Inport  Port=4
  Camber : Inport  Port=5
  MATLAB Function : MATLAB Function  TreatAsAtomicUnit=on
  Aligning Moment : Outport  VectorParamsAs1DForOutWhenUnconnected=off
  wires:
  MATLAB Function/1(Fyo) -> Aligning Moment/1
  Alpha/1 -> MATLAB Function/1(Alpha)
  Kappa/1 -> MATLAB Function/2(unused)
  Normal Forces/1 -> MATLAB Function/3(Fz)
  Pressure/1 -> MATLAB Function/4(Pi)
  Camber/1 -> MATLAB Function/5(Gam)

== system FRUCD_VehicleSim_Model_V0_1_0/Tire Force Evaluation/Lateral Force Evaluation/Cornering Coefficient Lookup ==
  Alpha : Inport
  Kappa : Inport  Port=2
  Normal Forces : Inport  Port=3
  Pressure : Inport  Port=4
  Camber : Inport  Port=5
  MATLAB Function : MATLAB Function  TreatAsAtomicUnit=on
  Lateral Forces : Outport  VectorParamsAs1DForOutWhenUnconnected=off
  wires:
  Camber/1 -> MATLAB Function/5(Gam)
  Pressure/1 -> MATLAB Function/4(Pi)
  Normal Forces/1 -> MATLAB Function/3(Fz)
  Kappa/1 -> MATLAB Function/2(unused)
  Alpha/1 -> MATLAB Function/1(Alpha)
  MATLAB Function/1(Fyo) -> Lateral Forces/1

== system FRUCD_VehicleSim_Model_V0_1_0/Tire Force Evaluation/Lateral Force Evaluation/Pure MF 6.1 Pacejka Model ==
  Alpha : Inport
  Kappa : Inport  Port=2
  Normal Forces : Inport  Port=3
  Pressure : Inport  Port=4
  Camber : Inport  Port=5
  MATLAB Function : MATLAB Function  TreatAsAtomicUnit=on
  Lateral Forces : Outport  VectorParamsAs1DForOutWhenUnconnected=off
  wires:
  MATLAB Function/1(Fyo) -> Lateral Forces/1
  Alpha/1 -> MATLAB Function/1(Alpha)
  Kappa/1 -> MATLAB Function/2(unused)
  Normal Forces/1 -> MATLAB Function/3(Fz)
  Pressure/1 -> MATLAB Function/4(Pi)
  Camber/1 -> MATLAB Function/5(Gam)

== system FRUCD_VehicleSim_Model_V0_1_0/Tire Force Evaluation/Longitudinal Force Evaluation/Cornering Coefficient Lookup ==
  Alpha : Inport
  Kappa : Inport  Port=2
  Normal Forces : Inport  Port=3
  Pressure : Inport  Port=4
  Camber : Inport  Port=5
  MATLAB Function : MATLAB Function  TreatAsAtomicUnit=on
  Longitudinal Forces : Outport  VectorParamsAs1DForOutWhenUnconnected=off
  wires:
  Camber/1 -> MATLAB Function/5(unused)
  Pressure/1 -> MATLAB Function/4(Pi)
  Normal Forces/1 -> MATLAB Function/3(Fz)
  Kappa/1 -> MATLAB Function/2(Kappa)
  Alpha/1 -> MATLAB Function/1(unused1)
  MATLAB Function/1(Fxo) -> Longitudinal Forces/1

== system FRUCD_VehicleSim_Model_V0_1_0/Tire Force Evaluation/Longitudinal Force Evaluation/Pure MF 6.1 Pacejka Model ==
  Alpha : Inport
  Kappa : Inport  Port=2
  Normal Forces : Inport  Port=3
  Pressure : Inport  Port=4
  Camber : Inport  Port=5
  MATLAB Function : MATLAB Function  TreatAsAtomicUnit=on
  Longitudinal Forces : Outport  VectorParamsAs1DForOutWhenUnconnected=off
  wires:
  MATLAB Function/1(Fxo) -> Longitudinal Forces/1
  Alpha/1 -> MATLAB Function/1(unused)
  Kappa/1 -> MATLAB Function/2(Kappa)
  Normal Forces/1 -> MATLAB Function/3(Fz)
  Pressure/1 -> MATLAB Function/4(Pi)
  Camber/1 -> MATLAB Function/5(Gam)

== system FRUCD_VehicleSim_Model_V0_1_0/Tire Force Evaluation/Overturning Moment Evaluation/Cornering Coefficient Lookup ==
  Alpha : Inport
  Kappa : Inport  Port=2
  Normal Forces : Inport  Port=3
  Pressure : Inport  Port=4
  Camber : Inport  Port=5
  MATLAB Function : MATLAB Function  TreatAsAtomicUnit=on
  Overturning Moment : Outport  VectorParamsAs1DForOutWhenUnconnected=off
  wires:
  Camber/1 -> MATLAB Function/5(Gam)
  Pressure/1 -> MATLAB Function/4(Pi)
  Normal Forces/1 -> MATLAB Function/3(Fz)
  Kappa/1 -> MATLAB Function/2(unused)
  Alpha/1 -> MATLAB Function/1(a)
  MATLAB Function/1(Fyo) -> Overturning Moment/1

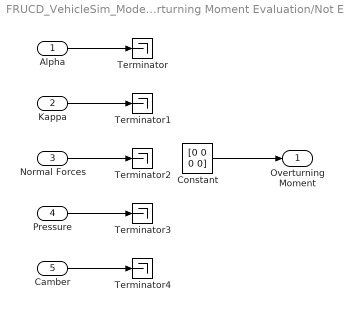
== system FRUCD_VehicleSim_Model_V0_1_0/Tire Force Evaluation/Overturning Moment Evaluation/Not Evaluated ==
  Alpha : Inport
  Kappa : Inport  Port=2
  Normal Forces : Inport  Port=3
  Pressure : Inport  Port=4
  Camber : Inport  Port=5
  Constant : Constant  Value=[0 0 0 0]
  Terminator{,1..4} (5 alike) : Terminator
  Overturning Moment : Outport  VectorParamsAs1DForOutWhenUnconnected=off
  wires:
  Kappa/1 -> Terminator1/1
  Alpha/1 -> Terminator/1
  Constant/1 -> Overturning Moment/1
  Normal Forces/1 -> Terminator2/1
  Pressure/1 -> Terminator3/1
  Camber/1 -> Terminator4/1

== system FRUCD_VehicleSim_Model_V0_1_0/Tire Force Evaluation/Overturning Moment Evaluation/Pure MF 6.1 Pacejka Model ==
  Alpha : Inport
  Kappa : Inport  Port=2
  Normal Forces : Inport  Port=3
  Pressure : Inport  Port=4
  Camber : Inport  Port=5
  MATLAB Function : MATLAB Function  TreatAsAtomicUnit=on
  Overturning Moment : Outport  VectorParamsAs1DForOutWhenUnconnected=off
  wires:
  MATLAB Function/1(Fyo) -> Overturning Moment/1
  Alpha/1 -> MATLAB Function/1(Alpha)
  Kappa/1 -> MATLAB Function/2(unused)
  Normal Forces/1 -> MATLAB Function/3(Fz)
  Pressure/1 -> MATLAB Function/4(Pi)
  Camber/1 -> MATLAB Function/5(Gam)

== system FRUCD_VehicleSim_Model_V0_1_0/Tire Force Evaluation/Rolling Resistance Evaluation/Cornering Coefficient Lookup ==
  Alpha : Inport
  Kappa : Inport  Port=2
  Normal Forces : Inport  Port=3
  Pressure : Inport  Port=4
  Camber : Inport  Port=5
  MATLAB Function : MATLAB Function  TreatAsAtomicUnit=on
  Rolling Resistance : Outport  VectorParamsAs1DForOutWhenUnconnected=off
  wires:
  Camber/1 -> MATLAB Function/5(Gam)
  Pressure/1 -> MATLAB Function/4(Pi)
  Normal Forces/1 -> MATLAB Function/3(Fz)
  Kappa/1 -> MATLAB Function/2(unused)
  Alpha/1 -> MATLAB Function/1(a)
  MATLAB Function/1(Fyo) -> Rolling Resistance/1

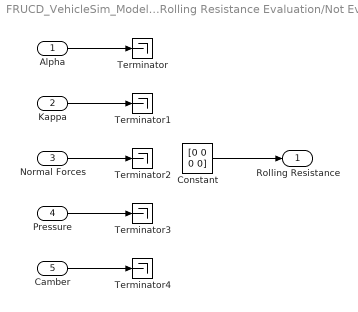
== system FRUCD_VehicleSim_Model_V0_1_0/Tire Force Evaluation/Rolling Resistance Evaluation/Not Evaluated ==
  Alpha : Inport
  Kappa : Inport  Port=2
  Normal Forces : Inport  Port=3
  Pressure : Inport  Port=4
  Camber : Inport  Port=5
  Constant : Constant  Value=[0 0 0 0]
  Terminator{,1..4} (5 alike) : Terminator
  Rolling Resistance : Outport  VectorParamsAs1DForOutWhenUnconnected=off
  wires:
  Kappa/1 -> Terminator1/1
  Alpha/1 -> Terminator/1
  Constant/1 -> Rolling Resistance/1
  Normal Forces/1 -> Terminator2/1
  Pressure/1 -> Terminator3/1
  Camber/1 -> Terminator4/1

== system FRUCD_VehicleSim_Model_V0_1_0/Tire Force Evaluation/Rolling Resistance Evaluation/Pure MF 6.1 Pacejka Model ==
  Alpha : Inport
  Kappa : Inport  Port=2
  Normal Forces : Inport  Port=3
  Pressure : Inport  Port=4
  Camber : Inport  Port=5
  MATLAB Function : MATLAB Function  TreatAsAtomicUnit=on
  Rolling Resistance : Outport  VectorParamsAs1DForOutWhenUnconnected=off
  wires:
  MATLAB Function/1(Fyo) -> Rolling Resistance/1
  Alpha/1 -> MATLAB Function/1(Alpha)
  Kappa/1 -> MATLAB Function/2(unused)
  Normal Forces/1 -> MATLAB Function/3(Fz)
  Pressure/1 -> MATLAB Function/4(Pi)
  Camber/1 -> MATLAB Function/5(Gam)

== matlab function FRUCD_VehicleSim_Model_V0_1_0/Chassis Dynamics/5DOF Sampo Model/MATLAB Function1 ==
  data: Delta input; FyR output; Fx input; Fy input
function FyR = LateralTireForces(Delta, Fx, Fy)

FyR = sum( Fy.*cosd(Delta) + Fx.*sind(Delta) );

== matlab function FRUCD_VehicleSim_Model_V0_1_0/Chassis Dynamics/5DOF Sampo Model/MATLAB Function ==
  data: Delta input; FxR output; Fx input; Fy input
function FxR = LongitudinalTireForces(Delta, Fx, Fy)

FxR = sum( Fx.*cosd(Delta) - Fy.*sind(Delta) );

== matlab function FRUCD_VehicleSim_Model_V0_1_0/Tire Force Evaluation/Lateral Force Evaluation/Cornering Coefficient Lookup/MATLAB Function ==
  data: Alpha input; Fyo output; unused input; Fz input; Pi input; Gam input; Parameter parameter
function Fyo = FyoLookup( Alpha, ~, Fz, Pi, Gam, Parameter)

dPi = (Pi - Parameter.Tire.Pio) ./ Parameter.Tire.Pio;

Kya = Parameter.Tire.p.K.y(1) .* Parameter.Tire.Fzo .* ( 1 + Parameter.Tire.p.P.y(1).*dPi ) .* ...
    ( 1 - Parameter.Tire.p.K.y(3).*abs(Gam) ) .* sin( Parameter.Tire.p.K.y(4) .* ...
    atan( (Fz./Parameter.Tire.Fzo) ./ ...
    ( ( Parameter.Tire.p.K.y(2) + Parameter.Tire.p.K.y(5).*Gam.^2 ) .* ( 1 + Parameter.Tire.p.P.y(2).*dPi ) ) ) );

Fyo = Kya.*Alpha;

== matlab function FRUCD_VehicleSim_Model_V0_1_0/Tire Force Evaluation/Lateral Force Evaluation/Pure MF 6.1 Pacejka Model/MATLAB Function ==
  data: Alpha input; Fyo output; unused input; Fz input; Pi input; Gam input; Parameter parameter
function Fyo = FyoMF6_1( Alpha, ~, Fz, Pi, Gam, Parameter)

dFz = (Fz - Parameter.Tire.Fzo) ./ Parameter.Tire.Fzo;
dPi = (Pi - Parameter.Tire.Pio) ./ Parameter.Tire.Pio;

Cy = Parameter.Tire.p.C.y(1);

Dy = (Parameter.Tire.p.D.y(1) + Parameter.Tire.p.D.y(2).*dFz) .* ...
    (1 + Parameter.Tire.p.P.y(3).*dPi + Parameter.Tire.p.P.y(4).*dPi.^2) .* ...
    (1 - Parameter.Tire.p.D.y(3).*Gam.^2).*Fz;

Kya = Parameter.Tire.p.K.y(1) .* Parameter.Tire.Fzo .* ( 1 + Parameter.Tire.p.P.y(1).*dPi ) .* ...
    ( 1 - Parameter.Tire.p.K.y(3).*abs(Gam) ) .* sin( Parameter.Tire.p.K.y(4) .* ...
    atan( (Fz./Parameter.Tire.Fzo) ./ ...
    ( ( Parameter.Tire.p.K.y(2) + Parameter.Tire.p.K.y(5).*Gam.^2 ) .* ( 1 + Parameter.Tire.p.P.y(2).*dPi ) ) ) );

Kyg0 =  Fz.*(Parameter.Tire.p.K.y(6) + Parameter.Tire.p.K.y(7).*dFz ) .* (1 + Parameter.Tire.p.P.y(5).*dPi );

By = Kya ./ ( Cy.*Dy );

Vyg = Fz.*(Parameter.Tire.p.V.y(3) + Parameter.Tire.p.V.y(4).*dFz ).*Gam;

Vy =  Fz.*(Parameter.Tire.p.V.y(1) + Parameter.Tire.p.V.y(2).*dFz ) + Vyg;

Hy = (Parameter.Tire.p.H.y(1) + Parameter.Tire.p.H.y(2).*dFz ) .* (Kyg0.*Gam - Vyg) ./ Kya;

Ey = ( Parameter.Tire.p.E.y(1) + Parameter.Tire.p.E.y(2).*dFz ) .* ...
    ( 1 + Parameter.Tire.p.E.y(5).*Gam.^2 - ...
    ( Parameter.Tire.p.E.y(3) + Parameter.Tire.p.E.y(4).*Gam ).*sign(Alpha + Hy) );

Fyo = Dy .* sin( Cy .* atan( (1-Ey) .* By.*(Alpha) + ...
    Ey.*atan( By.*(Alpha) ) ) );

%Fyo = Dy .* sin( Cy .* atan( (1-Ey) .* By.*(Alpha + Hy) + ...
%    Ey.*atan( By.*(Alpha + Hy) ) ) ) + Vy;

== matlab function FRUCD_VehicleSim_Model_V0_1_0/Tire Force Evaluation/Aligning Moment Evaluation/Cornering Coefficient Lookup/MATLAB Function ==
  data: a input; Fyo output; unused input; Fz input; Pi input; Gam input
function Fyo = FyoLookup( a, ~, Fz, Pi, Gam)

== matlab function FRUCD_VehicleSim_Model_V0_1_0/Tire Force Evaluation/Aligning Moment Evaluation/Pure MF 6.1 Pacejka Model/MATLAB Function ==
  data: Alpha input; Fyo output; unused input; Fz input; Pi input; Gam input
function Fyo = FyoMF6_1( Alpha, ~, Fz, Pi, Gam)

dFz = (Fz - Param.Tire.Fzo) ./ Param.Tire.Fzo;
dPi = (Pi - Param.Tire.Pio) ./ Param.Tire.Pio;

Cy = Param.Tire.p.C.y(1);

Dy = (Param.Tire.p.D.y(1) + Param.Tire.p.D.y(2).*dFz) .* ...
    (1 + Param.Tire.p.P.y(3).*dPi + Param.Tire.p.P.y(4).*dPi.^2) .* ...
    (1 - Param.Tire.p.D.y(3).*Gam.^2).*Fz;

Kya = Param.Tire.p.K.y(1) .* Param.Tire.Fzo .* ( 1 + Param.Tire.p.P.y(1).*dPi ) .* ...
    ( 1 - Param.Tire.p.K.y(3).*abs(Gam) ) .* sin( Param.Tire.p.K.y(4) .* ...
    atan( (Fz./Param.Tire.Fzo) ./ ...
    ( ( Param.Tire.p.K.y(2) + Param.Tire.p.K.y(5).*Gam.^2 ) .* ( 1 + Param.Tire.p.P.y(2).*dPi ) ) ) );

Kyg0 =  Fz.*(Param.Tire.p.K.y(6) + Param.Tire.p.K.y(7).*dFz ) .* (1 + Param.Tire.p.P.y(5).*dPi );

By = Kya ./ ( Cy.*Dy );

Vyg = Fz.*(Param.Tire.p.V.y(3) + Param.Tire.p.V.y(4).*dFz ).*Gam;

Vy =  Fz.*(Param.Tire.p.V.y(1) + Param.Tire.p.V.y(2).*dFz ) + Vyg;

Hy = (Param.Tire.p.H.y(1) + Param.Tire.p.H.y(2).*dFz ) .* (Kyg0.*Gam - Vyg) ./ Kya;

Ey = ( Param.Tire.p.E.y(1) + Param.Tire.p.E.y(2).*dFz ) .* ...
    ( 1 + Param.Tire.p.E.y(5).*Gam.^2 - ...
    ( Param.Tire.p.E.y(3) + Param.Tire.p.E.y(4).*Gam ).*sign(Alpha + Hy) );

Fyo = Dy .* sin( Cy .* atan( (1-Ey) .* By.*(Alpha + Hy) + ...
    Ey.*atan( By.*(Alpha + Hy) ) ) ) + Vy;

== matlab function FRUCD_VehicleSim_Model_V0_1_0/Tire Force Evaluation/Longitudinal Force Evaluation/Cornering Coefficient Lookup/MATLAB Function ==
  data: unused1 input; Fxo output; Kappa input; Fz input; Pi input; unused input; Parameter parameter
function Fxo = FxoLookup( ~, Kappa, Fz, Pi, ~, Parameter)

dFz = (Fz - Parameter.Tire.Fzo) ./ Parameter.Tire.Fzo;
dPi = (Pi - Parameter.Tire.Pio) ./ Parameter.Tire.Pio;

Kxk = Fz.*(Parameter.Tire.p.K.x(1) + Parameter.Tire.p.K.x(2).*dFz ) .* ...
    exp( Parameter.Tire.p.K.x(3) .* dFz ) .* ...
    (1 + Parameter.Tire.p.P.x(1).*dPi + Parameter.Tire.p.P.x(2).*dPi.^2);

Fxo = Kxk.*Kappa;

== matlab function FRUCD_VehicleSim_Model_V0_1_0/Tire Force Evaluation/Longitudinal Force Evaluation/Pure MF 6.1 Pacejka Model/MATLAB Function ==
  data: unused input; Fxo output; Kappa input; Fz input; Pi input; Gam input; Parameter parameter
function Fxo = FxoMF6_1( ~, Kappa, Fz, Pi, Gam, Parameter)

dFz = (Fz - Parameter.Tire.Fzo) ./ Parameter.Tire.Fzo;
dPi = (Pi - Parameter.Tire.Pio) ./ Parameter.Tire.Pio;

Cx = Parameter.Tire.p.C.x(1);

Dx = (Parameter.Tire.p.D.x(1) + Parameter.Tire.p.D.x(2).*dFz) .* ...
    (1 + Parameter.Tire.p.P.x(3).*dPi + Parameter.Tire.p.P.x(4).*dPi.^2) .* ...
    (1 - Parameter.Tire.p.D.x(3).*Gam.^2).*Fz;

Ex = ( Parameter.Tire.p.E.x(1) + Parameter.Tire.p.E.x(2).*dFz ...
    + Parameter.Tire.p.E.x(3).*dFz.^2 ) .* ( 1 - Parameter.Tire.p.E.x(4).*sign(Kappa) );

Kxk = Fz.*(Parameter.Tire.p.K.x(1) + Parameter.Tire.p.K.x(2).*dFz ) .* ...
    exp( Parameter.Tire.p.K.x(3) .* dFz ) .* ...
    (1 + Parameter.Tire.p.P.x(1).*dPi + Parameter.Tire.p.P.x(2).*dPi.^2);

Bx = Kxk ./ ( Cx.*Dx );

Vx = Fz.*(Parameter.Tire.p.V.x(1) + Parameter.Tire.p.V.x(2).*dFz );

Hx = Parameter.Tire.p.H.x(1) + Parameter.Tire.p.H.x(2).*dFz;

Fxo = Dx .* sin( Cx .* atan( (1-Ex) .* Bx.*(Kappa) + ...
    Ex.*atan( Bx.*(Kappa) ) ) );

%Fxo = Dx .* sin( Cx .* atan( (1-Ex) .* Bx.*(Kappa - Hx) + ...
%    Ex.*atan( Bx.*(Kappa - Hx) ) ) ) + Vx;

== matlab function FRUCD_VehicleSim_Model_V0_1_0/Tire Force Evaluation/Overturning Moment Evaluation/Cornering Coefficient Lookup/MATLAB Function ==
  data: a input; Fyo output; unused input; Fz input; Pi input; Gam input
function Fyo = FyoLookup( a, ~, Fz, Pi, Gam)

== matlab function FRUCD_VehicleSim_Model_V0_1_0/Tire Force Evaluation/Overturning Moment Evaluation/Pure MF 6.1 Pacejka Model/MATLAB Function ==
  data: Alpha input; Fyo output; unused input; Fz input; Pi input; Gam input
function Fyo = FyoMF6_1( Alpha, ~, Fz, Pi, Gam)

dFz = (Fz - Param.Tire.Fzo) ./ Param.Tire.Fzo;
dPi = (Pi - Param.Tire.Pio) ./ Param.Tire.Pio;

Cy = Param.Tire.p.C.y(1);

Dy = (Param.Tire.p.D.y(1) + Param.Tire.p.D.y(2).*dFz) .* ...
    (1 + Param.Tire.p.P.y(3).*dPi + Param.Tire.p.P.y(4).*dPi.^2) .* ...
    (1 - Param.Tire.p.D.y(3).*Gam.^2).*Fz;

Kya = Param.Tire.p.K.y(1) .* Param.Tire.Fzo .* ( 1 + Param.Tire.p.P.y(1).*dPi ) .* ...
    ( 1 - Param.Tire.p.K.y(3).*abs(Gam) ) .* sin( Param.Tire.p.K.y(4) .* ...
    atan( (Fz./Param.Tire.Fzo) ./ ...
    ( ( Param.Tire.p.K.y(2) + Param.Tire.p.K.y(5).*Gam.^2 ) .* ( 1 + Param.Tire.p.P.y(2).*dPi ) ) ) );

Kyg0 =  Fz.*(Param.Tire.p.K.y(6) + Param.Tire.p.K.y(7).*dFz ) .* (1 + Param.Tire.p.P.y(5).*dPi );

By = Kya ./ ( Cy.*Dy );

Vyg = Fz.*(Param.Tire.p.V.y(3) + Param.Tire.p.V.y(4).*dFz ).*Gam;

Vy =  Fz.*(Param.Tire.p.V.y(1) + Param.Tire.p.V.y(2).*dFz ) + Vyg;

Hy = (Param.Tire.p.H.y(1) + Param.Tire.p.H.y(2).*dFz ) .* (Kyg0.*Gam - Vyg) ./ Kya;

Ey = ( Param.Tire.p.E.y(1) + Param.Tire.p.E.y(2).*dFz ) .* ...
    ( 1 + Param.Tire.p.E.y(5).*Gam.^2 - ...
    ( Param.Tire.p.E.y(3) + Param.Tire.p.E.y(4).*Gam ).*sign(Alpha + Hy) );

Fyo = Dy .* sin( Cy .* atan( (1-Ey) .* By.*(Alpha + Hy) + ...
    Ey.*atan( By.*(Alpha + Hy) ) ) ) + Vy;

== matlab function FRUCD_VehicleSim_Model_V0_1_0/Tire Force Evaluation/Rolling Resistance Evaluation/Cornering Coefficient Lookup/MATLAB Function ==
  data: a input; Fyo output; unused input; Fz input; Pi input; Gam input
function Fyo = FyoLookup( a, ~, Fz, Pi, Gam)

== matlab function FRUCD_VehicleSim_Model_V0_1_0/Tire Force Evaluation/Rolling Resistance Evaluation/Pure MF 6.1 Pacejka Model/MATLAB Function ==
  data: Alpha input; Fyo output; unused input; Fz input; Pi input; Gam input
function Fyo = FyoMF6_1( Alpha, ~, Fz, Pi, Gam)

dFz = (Fz - Param.Tire.Fzo) ./ Param.Tire.Fzo;
dPi = (Pi - Param.Tire.Pio) ./ Param.Tire.Pio;

Cy = Param.Tire.p.C.y(1);

Dy = (Param.Tire.p.D.y(1) + Param.Tire.p.D.y(2).*dFz) .* ...
    (1 + Param.Tire.p.P.y(3).*dPi + Param.Tire.p.P.y(4).*dPi.^2) .* ...
    (1 - Param.Tire.p.D.y(3).*Gam.^2).*Fz;

Kya = Param.Tire.p.K.y(1) .* Param.Tire.Fzo .* ( 1 + Param.Tire.p.P.y(1).*dPi ) .* ...
    ( 1 - Param.Tire.p.K.y(3).*abs(Gam) ) .* sin( Param.Tire.p.K.y(4) .* ...
    atan( (Fz./Param.Tire.Fzo) ./ ...
    ( ( Param.Tire.p.K.y(2) + Param.Tire.p.K.y(5).*Gam.^2 ) .* ( 1 + Param.Tire.p.P.y(2).*dPi ) ) ) );

Kyg0 =  Fz.*(Param.Tire.p.K.y(6) + Param.Tire.p.K.y(7).*dFz ) .* (1 + Param.Tire.p.P.y(5).*dPi );

By = Kya ./ ( Cy.*Dy );

Vyg = Fz.*(Param.Tire.p.V.y(3) + Param.Tire.p.V.y(4).*dFz ).*Gam;

Vy =  Fz.*(Param.Tire.p.V.y(1) + Param.Tire.p.V.y(2).*dFz ) + Vyg;

Hy = (Param.Tire.p.H.y(1) + Param.Tire.p.H.y(2).*dFz ) .* (Kyg0.*Gam - Vyg) ./ Kya;

Ey = ( Param.Tire.p.E.y(1) + Param.Tire.p.E.y(2).*dFz ) .* ...
    ( 1 + Param.Tire.p.E.y(5).*Gam.^2 - ...
    ( Param.Tire.p.E.y(3) + Param.Tire.p.E.y(4).*Gam ).*sign(Alpha + Hy) );

Fyo = Dy .* sin( Cy .* atan( (1-Ey) .* By.*(Alpha + Hy) + ...
    Ey.*atan( By.*(Alpha + Hy) ) ) ) + Vy;

== matlab function FRUCD_VehicleSim_Model_V0_1_0/Chassis Dynamics/5DOF Sampo Model/MATLAB Function2 ==
  data: Delta input size=4; MzR output size=1; Fx input size=4; Fy input size=4; Parameter parameter
function MzR = YawTireMoments(Delta, Fx, Fy, Parameter)

MzR = Parameter.Chassis.TrackWidth(1)/2 * ( -Fx(1)*cosd( Delta(1) ) ) + ...
    Parameter.Chassis.a * ( Fx(1)*sind( Delta(1) ) ) + ...
    Parameter.Chassis.TrackWidth(1)/2 * ( Fy(1)*sind( Delta(1) ) ) + ...
    Parameter.Chassis.a * ( Fy(1)*cosd( Delta(1) ) ) + ...
    Parameter.Chassis.TrackWidth(1)/2 * ( Fx(2)*cosd( Delta(2) ) ) + ...
    Parameter.Chassis.a * ( Fx(2)*sind( Delta(2) ) ) + ...
    Parameter.Chassis.TrackWidth(1)/2 * ( -Fy(2)*sind( Delta(2) ) ) + ...
    Parameter.Chassis.a * ( Fy(2)*cosd( Delta(2) ) ) + ...
    Parameter.Chassis.TrackWidth(2)/2 * ( -Fx(3)*cosd( Delta(3) ) ) + ...
    Parameter.Chassis.b * ( -Fx(3)*sind( Delta(3) ) ) + ...
    Parameter.Chassis.TrackWidth(2)/2 * ( Fy(3)*sind( Delta(3) ) ) + ...
    Parameter.Chassis.b * ( -Fy(3)*cosd( Delta(3) ) ) + ...
    Parameter.Chassis.TrackWidth(2)/2 * ( Fx(4)*cosd( Delta(4) ) ) + ...
    Parameter.Chassis.b * ( -Fx(4)*sind( Delta(4) ) ) + ...
    Parameter.Chassis.TrackWidth(2)/2 * ( Fy(4)*sind( Delta(4) ) ) + ...
    Parameter.Chassis.b * ( -Fy(4)*cosd( Delta(4) ) );

== matlab function FRUCD_VehicleSim_Model_V0_1_0/Slip Estimation/Planar Geometry/MATLAB Function ==
  data: Delta input; Alpha output; Long input; Lat input; Yaw input; Parameter parameter
function Alpha = SlipAngleCalculation(Delta, Long, Lat, Yaw, Parameter)

Alpha = zeros(4,1);

Alpha(1) = Delta(1) - atan2d( (Lat + Parameter.Chassis.a*Yaw ), ...
    ( Long - (Parameter.Chassis.TrackWidth(1)/2)*Yaw ) );

Alpha(2) = Delta(2) - atan2d( (Lat + Parameter.Chassis.a*Yaw ), ...
    ( Long + (Parameter.Chassis.TrackWidth(1)/2)*Yaw ) );

Alpha(3) = Delta(3) - atan2d( (Lat - Parameter.Chassis.b*Yaw ), ...
    ( Long - (Parameter.Chassis.TrackWidth(2)/2)*Yaw ) );

Alpha(4) = Delta(4) - atan2d( (Lat - Parameter.Chassis.b*Yaw ), ...
    ( Long + (Parameter.Chassis.TrackWidth(2)/2)*Yaw ) );

== matlab function FRUCD_VehicleSim_Model_V0_1_0/Slip Estimation/Planar Geometry/MATLAB Function1 ==
  data: Alpha input; Omega input; Kappa output; Long input; Lat input; Yaw input; Parameter parameter
function Kappa = SlipRatioCalculation(Alpha, Omega, Long, Lat, Yaw, Parameter)

v = zeros(4,1);
Kappa = zeros(4,1);

v(1) = sqrt( ( Long - (Parameter.Chassis.TrackWidth(1)/2)*Yaw )^2 + ...
    (Lat + Parameter.Chassis.a*Yaw )^2 );
v(2) = sqrt( ( Long + (Parameter.Chassis.TrackWidth(1)/2)*Yaw )^2 + ...
    (Lat + Parameter.Chassis.a*Yaw )^2 );
v(3) = sqrt( ( Long - (Parameter.Chassis.TrackWidth(2)/2)*Yaw )^2 + ...
    (Lat - Parameter.Chassis.b*Yaw )^2 );
v(4) = sqrt( ( Long + (Parameter.Chassis.TrackWidth(2)/2)*Yaw )^2 + ...
    (Lat - Parameter.Chassis.b*Yaw )^2 );

Kappa(1) = ( Omega(1) .* Parameter.Tire.Re ) / ( v(1) .* cosd(Alpha(1)) ) - 1;  
Kappa(2) = ( Omega(2) .* Parameter.Tire.Re ) / ( v(2) .* cosd(Alpha(2)) ) - 1;  
Kappa(3) = ( Omega(3) .* Parameter.Tire.Re ) / ( v(3) .* cosd(Alpha(3)) ) - 1;  
Kappa(4) = ( Omega(4) .* Parameter.Tire.Re ) / ( v(4) .* cosd(Alpha(4)) ) - 1;

== matlab function FRUCD_VehicleSim_Model_V0_1_0/Chassis Dynamics/5DOF Sampo Model/MATLAB Function3 ==
  data: y_ddot input; Fz output [50..]; Parameter parameter
function Fz = SampoSteadyLateralTransfer(y_ddot, Parameter)
%% Assignment
g = Parameter.Mass.Gravity;

m_sf = Parameter.Mass.Sprung(1);
m_sr = Parameter.Mass.Sprung(2);
m_uf = Parameter.Mass.Unsprung(1);
m_ur = Parameter.Mass.Unsprung(2);

k_f = Parameter.Suspension.Roll.Stiffness(1);
k_r = Parameter.Suspension.Roll.Stiffness(2);

z_f = Parameter.Suspension.Roll.Center(1);
z_r = Parameter.Suspension.Roll.Center(2);

d_sf = Parameter.Suspension.Roll.Arm(1);
d_sr = Parameter.Suspension.Roll.Arm(2);

h_uf = Parameter.Mass.Height.Unsprung(1);
h_ur = Parameter.Mass.Height.Unsprung(2);

t_f = Parameter.Chassis.TrackWidth(1);
t_r = Parameter.Chassis.TrackWidth(2);

%% Weight Transfer
dFz = zeros(2,1);

dFz(1) = ( (k_f.*d_sf.*m_sf + k_f.*d_sr.*m_sr ) ./ (k_f+k_r) + ...
    z_f.*m_sf + h_uf.*m_uf ) .* y_ddot ./ t_f;

dFz(2) = ( (k_r.*d_sf.*m_sf + k_r.*d_sr.*m_sr ) ./ (k_f+k_r) + ...
    z_r.*m_sr + h_ur.*m_ur ) .* y_ddot ./ t_r;

%% Updating Tire Loads
Fz = zeros(4,1);

Fz(1) = (m_sf + m_uf)*g/2 - dFz(1);
Fz(2) = (m_sf + m_uf)*g/2 + dFz(1);

Fz(3) = (m_sr + m_ur)*g/2 - dFz(2);
Fz(4) = (m_sr + m_ur)*g/2 + dFz(2);
